simulink model "comparepidcontrollers"  (R2020b)
settings: Solver=FixedStepAuto  StartTime=0.0  StopTime=30  FixedStep=0.01  RelTol=1e-3
values from neighbouring files (symbols this model uses):
  C0 = 1/(C*Ce*(tauC+L/2))    (= 4.44444444444)    [comparacion_controladores.m]
  C1 = max(T,L/2)*C0    [comparacion_controladores.m]
  Cd = min(T,L/2)*Ce    [comparacion_controladores.m]
  Ce = 1    [comparacion_controladores.m]
  pidController = pidtune(G,'pidf')    [comparacion_controladores.m]
libraries: cstblocks x3, fuzblock x2
settings Model: Creator=The MathWorks, Inc.  LastModifiedBy=snopv
settings DebuggingCC: SymbolicDimsDataTypeCodeGenerationDiagnostic=none

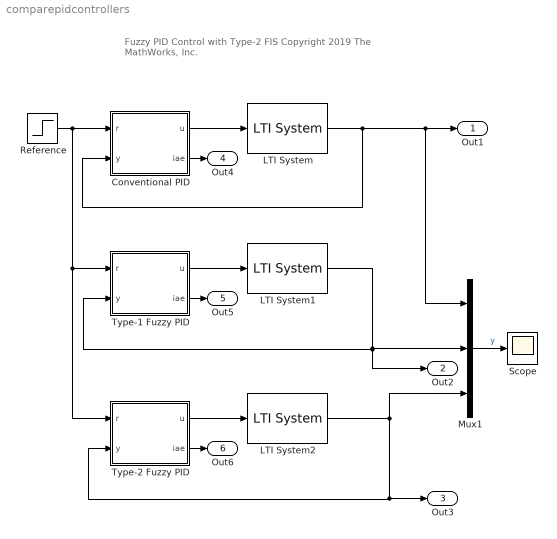
== system comparepidcontrollers ==
  note: Fuzzy PID Control with Type-2 FIS
      |
      | Copyright 2019 The MathWorks, Inc.
  Conventional PID : Subsystem
  LTI System : cstblocks/LTI System  sys=G  IC=[]
  LTI System1 : cstblocks/LTI System  sys=G  IC=[]
  LTI System2 : cstblocks/LTI System  sys=G  IC=[]
  Mux1 : Mux  Inputs=3
  Reference : Step  SampleTime=0
  Scope : Scope
  Type-1 Fuzzy PID : Subsystem
  Type-2 Fuzzy PID : Subsystem
  Out1 : Outport  VectorParamsAs1DForOutWhenUnconnected=off
  Out2 : Outport  Port=2  VectorParamsAs1DForOutWhenUnconnected=off
  Out3 : Outport  Port=3  VectorParamsAs1DForOutWhenUnconnected=off
  Out4 : Outport  Port=4  VectorParamsAs1DForOutWhenUnconnected=off
  Out5 : Outport  Port=5  VectorParamsAs1DForOutWhenUnconnected=off
  Out6 : Outport  Port=6  VectorParamsAs1DForOutWhenUnconnected=off
  wires:
  Reference/1 -> Type-2 Fuzzy PID/1(r), Type-1 Fuzzy PID/1(r), Conventional PID/1(r)
  Mux1/1 -> Scope/1  "y"
  LTI System/1 -> Conventional PID/2(y), Mux1/1, Out1/1
  Conventional PID/1(u) -> LTI System/1
  Type-1 Fuzzy PID/1(u) -> LTI System1/1
  LTI System1/1 -> Type-1 Fuzzy PID/2(y), Out2/1, Mux1/2
  Type-2 Fuzzy PID/1(u) -> LTI System2/1
  LTI System2/1 -> Type-2 Fuzzy PID/2(y), Out3/1, Mux1/3
  Conventional PID/2(iae) -> Out4/1
  Type-1 Fuzzy PID/2(iae) -> Out5/1
  Type-2 Fuzzy PID/2(iae) -> Out6/1

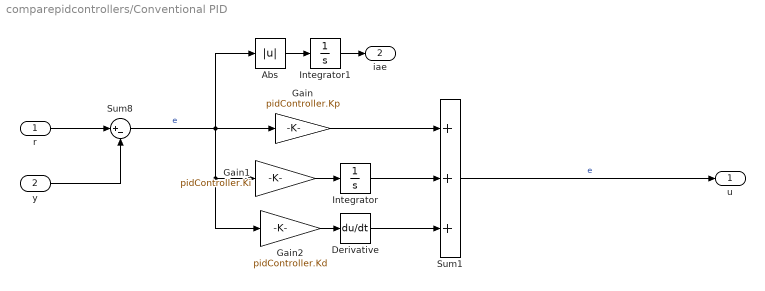
== system comparepidcontrollers/Conventional PID ==
  r : Inport
  y : Inport  Port=2
  Abs : Abs
  Derivative : Derivative  CoefficientInTFapproximation=pidController.Tf
  Gain : Gain  Gain=pidController.Kp
  Gain1 : Gain  Gain=pidController.Ki
  Gain2 : Gain  Gain=pidController.Kd
  Integrator : Integrator
  Integrator1 : Integrator
  Sum1 : Sum  Inputs=+++
  Sum8 : Sum  Inputs=|+-
  u : Outport  VectorParamsAs1DForOutWhenUnconnected=off
  iae : Outport  Port=2  VectorParamsAs1DForOutWhenUnconnected=off
  wires:
  r/1 -> Sum8/1
  y/1 -> Sum8/2
  Sum1/1 -> u/1  "e"
  Sum8/1 -> Abs/1, Gain2/1, Gain1/1, Gain/1  "e"
  Gain/1 -> Sum1/1
  Gain1/1 -> Integrator/1
  Integrator/1 -> Sum1/2
  Gain2/1 -> Derivative/1
  Derivative/1 -> Sum1/3
  Abs/1 -> Integrator1/1
  Integrator1/1 -> iae/1

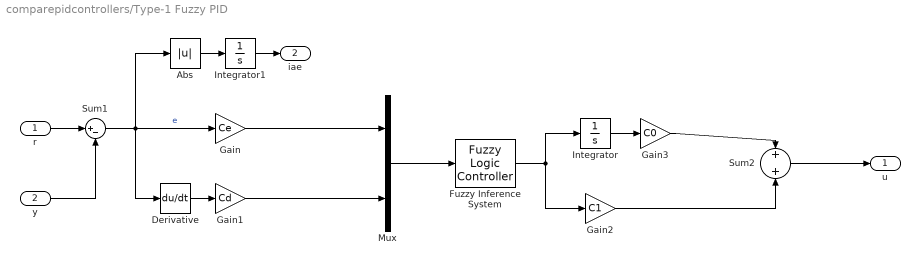
== system comparepidcontrollers/Type-1 Fuzzy PID ==
  r : Inport
  y : Inport  Port=2
  Abs : Abs
  Derivative : Derivative  CoefficientInTFapproximation=1
  Fuzzy Inference System : fuzblock/Fuzzy Logic  Controller  FIS=fis1  OutputSampleNumber=101  DataType=double  FuzzifiedInputs=off  RuleFiringStrengths=off  RuleOutputs=off  AggregatedOutputs=off  SimulateUsing=Code generation  OutOfRangeInputValueMessage=none  NoRuleFiredMessage=none  EmptyOutputFuzzySetMessage=none
  Gain : Gain  Gain=Ce
  Gain1 : Gain  Gain=Cd
  Gain2 : Gain  Gain=C1
  Gain3 : Gain  Gain=C0
  Integrator : Integrator
  Integrator1 : Integrator
  Mux : Mux  Inputs=2
  Sum1 : Sum  Inputs=|+-
  Sum2 : Sum  Inputs=+|+
  u : Outport  VectorParamsAs1DForOutWhenUnconnected=off
  iae : Outport  Port=2  VectorParamsAs1DForOutWhenUnconnected=off
  wires:
  Sum1/1 -> Abs/1, Derivative/1, Gain/1  "e"
  Mux/1 -> Fuzzy Inference System/1
  Fuzzy Inference System/1 -> Gain2/1, Integrator/1
  r/1 -> Sum1/1
  y/1 -> Sum1/2
  Sum2/1 -> u/1
  Derivative/1 -> Gain1/1
  Integrator/1 -> Gain3/1
  Gain/1 -> Mux/1
  Gain1/1 -> Mux/2
  Gain2/1 -> Sum2/2
  Gain3/1 -> Sum2/1
  Abs/1 -> Integrator1/1
  Integrator1/1 -> iae/1

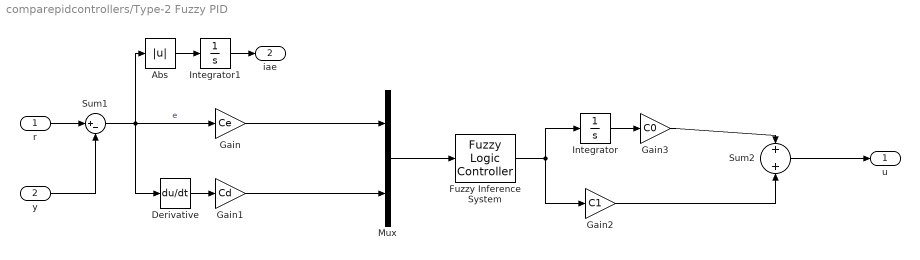
== system comparepidcontrollers/Type-2 Fuzzy PID ==
  r : Inport
  y : Inport  Port=2
  Abs : Abs
  Derivative : Derivative  CoefficientInTFapproximation=1
  Fuzzy Inference System : fuzblock/Fuzzy Logic  Controller  FIS=fis2  OutputSampleNumber=101  DataType=double  FuzzifiedInputs=off  RuleFiringStrengths=off  RuleOutputs=off  AggregatedOutputs=off  SimulateUsing=Code generation  OutOfRangeInputValueMessage=none  NoRuleFiredMessage=none  EmptyOutputFuzzySetMessage=none
  Gain : Gain  Gain=Ce
  Gain1 : Gain  Gain=Cd
  Gain2 : Gain  Gain=C1
  Gain3 : Gain  Gain=C0
  Integrator : Integrator
  Integrator1 : Integrator
  Mux : Mux  Inputs=2
  Sum1 : Sum  Inputs=|+-
  Sum2 : Sum  Inputs=+|+
  u : Outport  VectorParamsAs1DForOutWhenUnconnected=off
  iae : Outport  Port=2  VectorParamsAs1DForOutWhenUnconnected=off
  wires:
  Gain3/1 -> Sum2/1
  Gain2/1 -> Sum2/2
  Gain1/1 -> Mux/2
  Gain/1 -> Mux/1
  Integrator/1 -> Gain3/1
  Derivative/1 -> Gain1/1
  Sum2/1 -> u/1
  y/1 -> Sum1/2
  r/1 -> Sum1/1
  Fuzzy Inference System/1 -> Integrator/1, Gain2/1
  Mux/1 -> Fuzzy Inference System/1
  Sum1/1 -> Abs/1, Gain/1, Derivative/1  "e"
  Integrator1/1 -> iae/1
  Abs/1 -> Integrator1/1
